simulink model "plantaClosedLoopPID"  (R2022b)
settings: Solver=VariableStepAuto  StartTime=0.0  StopTime=100  MaxStep=0.01  RelTol=1e-3
undefined symbols (not defined in the file): d1, d2, DZ, I, km, miu, wb, wcp, wm
libraries: slpidlib x2
settings Model: Creator=felip  LastModifiedBy=felip

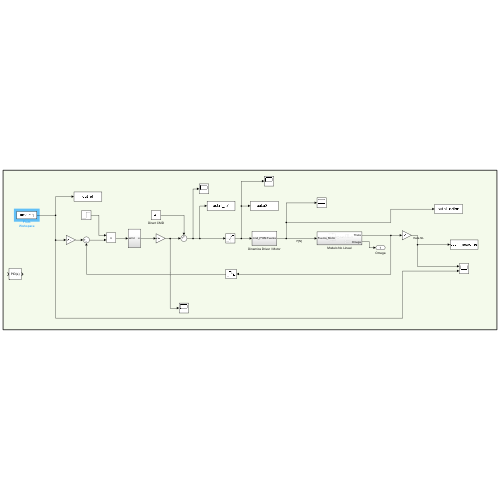
[thumbnail: Simulink's stored preview of the top-level diagram]
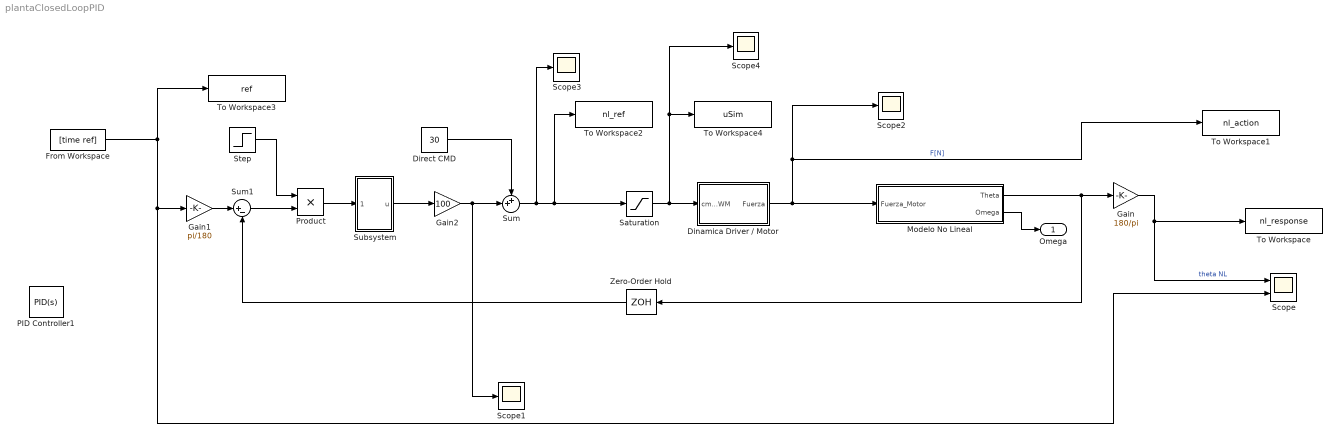
== system plantaClosedLoopPID ==
  Dinamica Driver / Motor : Subsystem
  Direct CMD : Constant  Value=30
  From Workspace : FromWorkspace  VariableName=[time ref]  SampleTime=2.5e-3
  Gain : Gain  Gain=180/pi
  Gain1 : Gain  Gain=pi/180
  Gain2 : Gain  Gain=100
  Modelo No Lineal : Subsystem
  PID Controller1 : slpidlib/PID Controller  Controller=PID  Form=Parallel  TimeDomain=Continuous-time  UseExternalTs=off  SampleTime=-1  IntegratorMethod=Forward Euler  FilterMethod=Forward Euler  ControllerParametersSource=internal  P=0.4  I=0.645  UseKiTs=off  D=0.018  N=100  UseFilter=on  TunerSelectOption=Transfer Function Based (PID Tuner App)  InitialConditionSource=internal  InitialConditionForIntegrator=0  InitialConditionForFilter=0  DifferentiatorICPrevScaledInput=0  ExternalReset=none  TrackingMode=off  Kt=1  LimitOutput=off  SatLimitsSource=internal  UpperSaturationLimit=inf  LowerSaturationLimit=-inf  LinearizeAsGain=on  AntiWindupMode=none  Kb=1  LimitIntegrator=off  UpperIntegratorSaturationLimit=inf  LowerIntegratorSaturationLimit=-inf  POutMin=[]  POutMax=[]  IOutMin=[]  IOutMax=[]  DOutMin=[]  DOutMax=[]  NOutMin=[]  NOutMax=[]  SumOutMin=[]  SumOutMax=[]  SaturationOutMin=[]  SaturationOutMax=[]  PParamMin=[]  PParamMax=[]  IParamMin=[]  IParamMax=[]  DParamMin=[]  DParamMax=[]  NParamMin=[]  NParamMax=[]  KbParamMin=[]  KbParamMax=[]  KtParamMin=[]  KtParamMax=[]  KbOutMin=[]  KbOutMax=[]  KtOutMin=[]  KtOutMax=[]  IntegratorOutMin=[]  IntegratorOutMax=[]  FilterOutMin=[]  FilterOutMax=[]  SumI1OutMin=[]  SumI1OutMax=[]  SumI2OutMin=[]  SumI2OutMax=[]  SumI3OutMin=[]  SumI3OutMax=[]  SumI4OutMin=[]  SumI4OutMax=[]  SumDOutMin=[]  SumDOutMax=[]  DifferentiatorOutMin=[]  DifferentiatorOutMax=[]  FilterDiffOutCoefMin=[]  FilterDiffOutCoefMax=[]  ReciprocalOutMin=[]  ReciprocalOutMax=[]  SumDenOutMin=[]  SumDenOutMax=[]  SumNumOutMin=[]  SumNumOutMax=[]  DivideOutMin=[]  DivideOutMax=[]  UdiffTsProdOutMin=[]  UdiffTsProdOutMax=[]  NTsProdOutMin=[]  NTsProdOutMax=[]  UintegralTsProdOutMin=[]  UintegralTsProdOutMax=[]  UngainTsProdOutMin=[]  UngainTsProdOutMax=[]  ClampingZeroOutDataTypeStr=Inherit: Inherit via back propagation  ClampingZeroOutMin=[]  ClampingZeroOutMax=[]  FilterDenConstantOutDataTypeStr=Inherit: Inherit via back propagation  FilterDenConstantOutMin=[]  FilterDenConstantOutMax=[]  PCopyOutDataTypeStr=Inherit: Inherit via back propagation  PCopyOutMin=[]  PCopyOutMax=[]  NCopyOutDataTypeStr=Inherit: Inherit via back propagation  NCopyOutMin=[]  NCopyOutMax=[]  IntegratorContinuousStateAttributes=''  IntegratorStateMustResolveToSignalObject=off  IntegratorRTWStateStorageClass=Auto  FilterContinuousStateAttributes=''  FilterStateMustResolveToSignalObject=off  FilterRTWStateStorageClass=Auto  ParallelPVariant=InternalParameters  IdealPVariant=Disabled  IVariant=InternalParameters  DVariant=InternalParameters  IntegratorVariant=Continuous  SatVariant=Disabled  AWVariant=Passthrough  PCopyVariant=Disabled  TRVariant=Disabled  FdbkBlocksVariant=Forward  IdealPFdbkVariant=Disabled  SatFdbkVariant=Disabled  DerivativeFilterVariant=ContFilter  NVariant=InternalParameters  NCopyVariant=Disabled  FilterICVariant=InternalICsFilter  IntegratorICVariant=InternalICs  ExternalResetVariant=Disabled  TRSumVariant=Passthrough  SumFdbkVariant=Disabled  SumVariant=Sum_PID  TsampFilterVariant=InternalTs  TsampNgainVariant=Passthrough  TsampIntegralVariant=Passthrough  ExternalSaturationOutDataTypeStr=Inherit: Same as second input
  Product : Product
  Saturation : Saturate  UpperLimit=100  LowerLimit=0
  Scope : Scope  NumInputPorts=2
  Scope{1..4} (4 alike) : Scope
  Step : Step  Time=5  SampleTime=0
  Subsystem : Subsystem
  Sum : Sum  Inputs=++|
  Sum1 : Sum  Inputs=|+-
  To Workspace : ToWorkspace  VariableName=nl_response  SaveFormat=Timeseries  SampleTime=-1
  To Workspace1 : ToWorkspace  VariableName=nl_action  SaveFormat=Timeseries  SampleTime=-1
  To Workspace2 : ToWorkspace  VariableName=nl_ref  SaveFormat=Timeseries  SampleTime=-1
  To Workspace3 : ToWorkspace  VariableName=ref  SaveFormat=Timeseries  SampleTime=-1
  To Workspace4 : ToWorkspace  VariableName=uSim  SaveFormat=Timeseries  SampleTime=-1
  Zero-Order Hold : ZeroOrderHold  SampleTime=2.5e-3
  Omega : Outport
  wires:
  Dinamica Driver / Motor/1(Fuerza) -> Scope2/1, To Workspace1/1, Modelo No Lineal/1(Fuerza_Motor)  "F[N]"
  Modelo No Lineal/1(Theta) -> Gain/1, Zero-Order Hold/1
  Modelo No Lineal/2(Omega) -> Omega/1
  Direct CMD/1 -> Sum/1
  Gain/1 -> Scope/1, To Workspace/1  "theta NL"
  Sum/1 -> Scope3/1, Saturation/1, To Workspace2/1
  Saturation/1 -> To Workspace4/1, Scope4/1, Dinamica Driver / Motor/1(cmd_PWM)
  Gain1/1 -> Sum1/1
  Step/1 -> Product/1
  Gain2/1 -> Scope1/1, Sum/2
  Zero-Order Hold/1 -> Sum1/2
  Subsystem/1(u) -> Gain2/1
  Product/1 -> Subsystem/1(error)
  Sum1/1 -> Product/2
  From Workspace/1 -> Scope/2, Gain1/1, To Workspace3/1

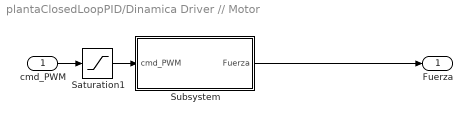
== system plantaClosedLoopPID/Dinamica Driver // Motor ==
  cmd_PWM : Inport
  Saturation1 : Saturate  UpperLimit=100
  Subsystem : Subsystem
  Fuerza : Outport
  wires:
  cmd_PWM/1 -> Saturation1/1
  Saturation1/1 -> Subsystem/1(cmd_PWM)
  Subsystem/1(Fuerza) -> Fuerza/1

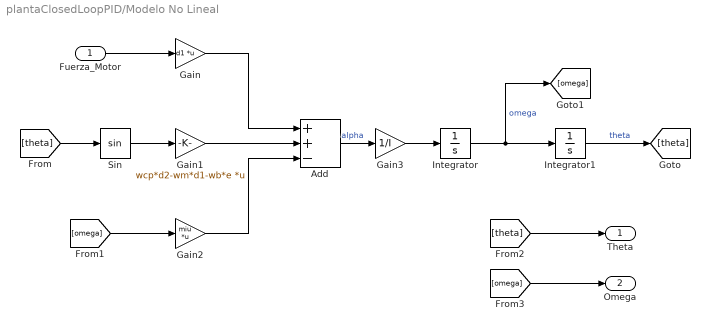
== system plantaClosedLoopPID/Modelo No Lineal ==
  Fuerza_Motor : Inport
  Add : Sum  Inputs=++-
  Gain : Gain  Gain=d1  Multiplication=Matrix(K*u)
  Gain1 : Gain  Gain=wcp*d2-wm*d1-wb*e  Multiplication=Matrix(K*u)
  Gain2 : Gain  Gain=miu  Multiplication=Matrix(K*u)
  Gain3 : Gain  Gain=1/I
  Integrator : Integrator
  Integrator1 : Integrator
  Sin : Trigonometry
  Theta : Outport
  Omega : Outport  Port=2
  wires:
  [omega] -> Omega/1
  Gain1/1 -> Add/2
  Integrator/1 -> [omega], Integrator1/1  "omega"
  Fuerza_Motor/1 -> Gain/1
  Integrator1/1 -> [theta]  "theta"
  Gain2/1 -> Add/3
  Gain/1 -> Add/1
  Add/1 -> Gain3/1  "alpha"
  [theta] -> Sin/1
  [omega] -> Gain2/1
  [theta] -> Theta/1
  Sin/1 -> Gain1/1
  Gain3/1 -> Integrator/1

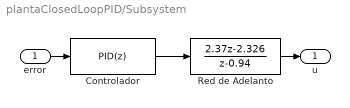
== system plantaClosedLoopPID/Subsystem ==
  error : Inport
  Controlador : slpidlib/PID Controller  Controller=PID  Form=Parallel  TimeDomain=Discrete-time  UseExternalTs=off  SampleTime=0.0025  IntegratorMethod=Forward Euler  FilterMethod=Forward Euler  ControllerParametersSource=internal  P=0.4  I=0.65  UseKiTs=off  D=0.018  N=100  UseFilter=off  TunerSelectOption=Transfer Function Based (PID Tuner App)  InitialConditionSource=internal  InitialConditionForIntegrator=0  InitialConditionForFilter=0  DifferentiatorICPrevScaledInput=0  ExternalReset=none  TrackingMode=off  Kt=1  LimitOutput=off  SatLimitsSource=internal  UpperSaturationLimit=inf  LowerSaturationLimit=-inf  LinearizeAsGain=off  AntiWindupMode=none  Kb=1  LimitIntegrator=off  UpperIntegratorSaturationLimit=inf  LowerIntegratorSaturationLimit=-inf  POutMin=[]  POutMax=[]  IOutMin=[]  IOutMax=[]  DOutMin=[]  DOutMax=[]  NOutMin=[]  NOutMax=[]  SumOutMin=[]  SumOutMax=[]  SaturationOutMin=[]  SaturationOutMax=[]  PParamMin=[]  PParamMax=[]  IParamMin=[]  IParamMax=[]  DParamMin=[]  DParamMax=[]  NParamMin=[]  NParamMax=[]  KbParamMin=[]  KbParamMax=[]  KtParamMin=[]  KtParamMax=[]  KbOutMin=[]  KbOutMax=[]  KtOutMin=[]  KtOutMax=[]  IntegratorOutMin=[]  IntegratorOutMax=[]  FilterOutMin=[]  FilterOutMax=[]  SumI1OutMin=[]  SumI1OutMax=[]  SumI2OutMin=[]  SumI2OutMax=[]  SumI3OutMin=[]  SumI3OutMax=[]  SumI4OutMin=[]  SumI4OutMax=[]  SumDOutMin=[]  SumDOutMax=[]  DifferentiatorOutMin=[]  DifferentiatorOutMax=[]  FilterDiffOutCoefMin=[]  FilterDiffOutCoefMax=[]  ReciprocalOutMin=[]  ReciprocalOutMax=[]  SumDenOutMin=[]  SumDenOutMax=[]  SumNumOutMin=[]  SumNumOutMax=[]  DivideOutMin=[]  DivideOutMax=[]  UdiffTsProdOutMin=[]  UdiffTsProdOutMax=[]  NTsProdOutMin=[]  NTsProdOutMax=[]  UintegralTsProdOutMin=[]  UintegralTsProdOutMax=[]  UngainTsProdOutMin=[]  UngainTsProdOutMax=[]  ClampingZeroOutDataTypeStr=Inherit: Inherit via back propagation  ClampingZeroOutMin=[]  ClampingZeroOutMax=[]  FilterDenConstantOutDataTypeStr=Inherit: Inherit via back propagation  FilterDenConstantOutMin=[]  FilterDenConstantOutMax=[]  PCopyOutDataTypeStr=Inherit: Inherit via back propagation  PCopyOutMin=[]  PCopyOutMax=[]  NCopyOutDataTypeStr=Inherit: Inherit via back propagation  NCopyOutMin=[]  NCopyOutMax=[]  IntegratorContinuousStateAttributes=''  IntegratorStateMustResolveToSignalObject=off  IntegratorRTWStateStorageClass=Auto  FilterContinuousStateAttributes=''  FilterStateMustResolveToSignalObject=off  FilterRTWStateStorageClass=Auto  ParallelPVariant=InternalParameters  IdealPVariant=Disabled  IVariant=InternalParameters  DVariant=InternalParameters  IntegratorVariant=Discrete  SatVariant=Disabled  AWVariant=Passthrough  PCopyVariant=Disabled  TRVariant=Disabled  FdbkBlocksVariant=Forward  IdealPFdbkVariant=Disabled  SatFdbkVariant=Disabled  DerivativeFilterVariant=Differentiator  NVariant=Passthrough  NCopyVariant=Disabled_SignalSpec  FilterICVariant=InternalICsDifferentiator  IntegratorICVariant=InternalICs  ExternalResetVariant=Disabled  TRSumVariant=Passthrough  SumFdbkVariant=Disabled  SumVariant=Sum_PID  TsampFilterVariant=InternalTs  TsampNgainVariant=Passthrough  TsampIntegralVariant=Passthrough  ExternalSaturationOutDataTypeStr=Inherit: Same as second input
      settings: LibrarySourceBlock=simulink/Discrete/Discrete PID Controller
  Red de Adelanto : DiscreteTransferFcn  Numerator=[2.37 -2.326]  Denominator=[1 -0.94]
  u : Outport
  wires:
  Controlador/1 -> Red de Adelanto/1
  Red de Adelanto/1 -> u/1
  error/1 -> Controlador/1

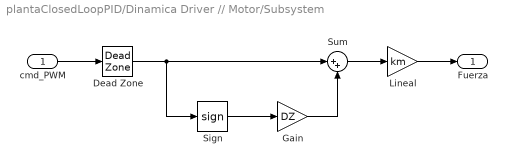
== system plantaClosedLoopPID/Dinamica Driver // Motor/Subsystem ==
  cmd_PWM : Inport
  Dead Zone : DeadZone  LowerValue=-DZ  UpperValue=DZ
  Gain : Gain  Gain=DZ
  Lineal : Gain  Gain=km
  Sign : Signum
  Sum : Sum  Inputs=|++
  Fuerza : Outport
  wires:
  cmd_PWM/1 -> Dead Zone/1
  Dead Zone/1 -> Sum/1, Sign/1
  Sum/1 -> Lineal/1
  Sign/1 -> Gain/1
  Gain/1 -> Sum/2
  Lineal/1 -> Fuerza/1
